simulink model "comprehensive_model_with_rocks_trial"  (R2019a)
settings: Solver=FixedStepAuto  StartTime=0.0  StopTime=15  FixedStep=0.001  RelTol=1e-3
PreLoadFcn:
  | load('tumbleweed_constants.mat')
values from neighbouring files (symbols this model uses):
  Ar = 0.785398163397    [tumbleweed_constants.mat]
  CD = 0.8    [tumbleweed_constants.mat]
  d = 0.65    [tumbleweed_constants.mat]
  g = 9.81    [tumbleweed_constants.mat]
  Ixx = 1.29    [tumbleweed_constants.mat]
  Iyy = 1.29    [tumbleweed_constants.mat]
  Izz = 1.29    [tumbleweed_constants.mat]
  m = 1    [tumbleweed_constants.mat]
  maxr = 0.45    [tumbleweed_constants.mat]
  mf = 14    [tumbleweed_constants.mat]
  minr = 0.2    [tumbleweed_constants.mat]
  mu0 = 0.02    [tumbleweed_constants.mat]
  muk = 0.5    [tumbleweed_constants.mat]
  must = 0.8    [tumbleweed_constants.mat]
  R = cylR*ones(size(Theta,1),size(Theta,2))    [d3_animate.m]    (also in tumbleweed_constants.mat = 0.5)
  rest_coeff = 0.6    [tumbleweed_constants.mat]
  rho = 1.2    [tumbleweed_constants.mat]
  ts = 0.5    [tumbleweed_constants.mat]
  v_thres = 0.0001    [tumbleweed_constants.mat]
  vmax = 0.2    [tumbleweed_constants.mat]
  YY = 50    [tumbleweed_constants.mat]
libraries: simulink x2
(part 9 of 9)

== matlab function comprehensive_model_with_rocks_trial/bouncing_model1/onsurface_model/Subsystem/MATLAB Function2 ==
  data: A21 output size=[3, 3]; t input; states input; u input; O_c_A input; O_w_A input; O_v_AO input; FW input; par_diffs input; flag input; A22 output size=[3, 3]; B2 output size=3; OalA_coeffs output size=[3,3]; OalA_consts output size=3; R parameter; g parameter; Ixx parameter; Iyy parameter; Izz parameter; m parameter; mf parameter; mu0 parameter; must parameter; d parameter; YY parameter; muk parameter; v_thres parameter
function [A21, A22, B2, OalA_coeffs, OalA_consts] = dynamics_mat_gen(t, states,u, O_c_A, O_w_A, O_v_AO, FW, par_diffs,flag, R, g, Ixx, Iyy, Izz, m, mf, mu0, must, d, YY, muk, v_thres)

y = states;
I_T = [Ixx,0,0;0,Iyy,0;0,0,Izz]; 
r_m1T = [u(1);0;0]; T_v_m1T = [u(7);0;0]; T_a_m1T = [u(13);0;0];
r_m2T = [u(2);0;0]; T_v_m2T = [u(8);0;0]; T_a_m2T = [u(14);0;0];
r_m3T = [0;u(3);0]; T_v_m3T = [0;u(9);0]; T_a_m3T = [0;u(15);0];
r_m4T = [0;u(4);0]; T_v_m4T = [0;u(10);0]; T_a_m4T = [0;u(16);0];
r_m5T = [0;0;u(5)]; T_v_m5T = [0;0;u(11)]; T_a_m5T = [0;0;u(17)];
r_m6T = [0;0;u(6)]; T_v_m6T = [0;0;u(12)]; T_a_m6T = [0;0;u(18)];
r_CMT = m*(r_m1T + r_m2T + r_m3T + r_m4T + r_m5T + r_m6T)/(6*m+mf);
T_v_CMT = m*(T_v_m1T + T_v_m2T + T_v_m3T + T_v_m4T + T_v_m5T + T_v_m6T)/(6*m+mf);
T_a_CMT = m*(T_a_m1T + T_a_m2T + T_a_m3T + T_a_m4T + T_a_m5T + T_a_m6T)/(6*m+mf);
r_CMTx = Vx(r_CMT);r_m1Tx = Vx(r_m1T);r_m2Tx = Vx(r_m2T);r_m3Tx = Vx(r_m3T);
r_m4Tx = Vx(r_m4T);r_m5Tx = Vx(r_m5T);r_m6Tx = Vx(r_m6T);
q0 = y(10);q1=y(11);q2=y(12);q3=y(13);
T_c_O = [q0^2 + q1^2 - q2^2 - q3^2, 2*(q1*q2 + q0*q3), 2*(q1*q3 - q0*q2);...
       2*(q1*q2 - q0*q3), q0^2 - q1^2 + q2^2 - q3^2, 2*(q2*q3 + q0*q1);...
       2*(q1*q3 + q0*q2), 2*(q2*q3 - q0*q1), q0^2 - q1^2 - q2^2 + q3^2];
O_c_T = T_c_O.';
T_c_A = T_c_O*O_c_A;
A_c_O = transpose(O_c_A);
A_c_T = T_c_A';
r_AT = [0;0;-R]; r_TA = [0;0;R]; r_ATx = Vx(r_AT); r_TAx = Vx(r_TA);

O_w_T = [y(1);y(2);y(3)];
A_w_T = O_w_T - T_c_A*O_w_A;
O_w_Tx = Vx(O_w_T);
O_w_Ax = Vx(O_w_A);

O_vel_TO = A_c_O*O_v_AO + cross(O_w_A, r_TA);
u_TO = O_vel_TO(1);
v_TO = O_vel_TO(2);
w_TO = O_vel_TO(3);

%mu0 =0.02;% 0.02;
murr = mu0*tanh(sqrt(u_TO^2 + v_TO^2 + w_TO^2)/v_thres); 
roll_rest_coeff = [1,0,-murr*u_TO/sqrt(u_TO^2 + v_TO^2);0,1,-murr*v_TO/sqrt(u_TO^2 + v_TO^2);0,0,1];
FG = [0;0;-(mf+6*m)*g];
FGA = A_c_O*FG;
FR  = -murr*norm(FGA'*[0;0;1])*[u_TO; v_TO; w_TO]/sqrt(u_TO^2 + v_TO^2 + w_TO^2);

eps = 0.025;
N = norm(FGA'*[0;0;1]);
f = 0.5;%0.5;
OwTz = (A_c_T*O_w_T)'*[0;0;1];
if(abs(OwTz) <= 1e-4)
    MzT = [0;0;0];
else
MzT = [0;0;-3*pi*N*f*eps*OwTz/(16*norm(OwTz))];%-mu*N*[0;0;1];
end


x_dot = O_v_AO(1);
y_dot = O_v_AO(2);
z_dot = O_v_AO(3);

fx = par_diffs(1);
fy = par_diffs(2);
fz = par_diffs(3);
fxx = par_diffs(4);
fxy = par_diffs(5);
fxz = par_diffs(6);
fyy = par_diffs(7);
fyz = par_diffs(8);
fzz = par_diffs(9);
fxxx = par_diffs(10);
fxxy = par_diffs(11);
fxxz = par_diffs(12);
fxyy = par_diffs(13);
fxyz = par_diffs(14);
fxzz = par_diffs(15);
fyyy = par_diffs(16);
fyyz = par_diffs(17);
fyzz = par_diffs(18);
fzzz = par_diffs(19);






if flag == 1
OalA_coeffs = ...
[(-(fx*fxy - fxx*fy)/((fx^2 + fy^2)^(1/2)*(fx^2 + fy^2 + fz^2)^(1/2))),                               (-(fx*fyy - fxy*fy)/((fx^2 + fy^2)^(1/2)*(fx^2 + fy^2 + fz^2)^(1/2))),                                     (-(fx*fyz - fxz*fy)/((fx^2 + fy^2)^(1/2)*(fx^2 + fy^2 + fz^2)^(1/2)));...
 (-(fxz*fx^2 - fxx*fz*fx + fxz*fy^2 - fxy*fz*fy)/((fx^2 + fy^2)^(1/2)*(fx^2 + fy^2 + fz^2))),          (-(fyz*fx^2 - fxy*fz*fx + fyz*fy^2 - fyy*fz*fy)/((fx^2 + fy^2)^(1/2)*(fx^2 + fy^2 + fz^2))),               (-(fzz*fx^2 - fxz*fz*fx + fzz*fy^2 - fyz*fz*fy)/((fx^2 + fy^2)^(1/2)*(fx^2 + fy^2 + fz^2)));...
 ((fz*(fx*fxy - fxx*fy))/((fx^2 + fy^2)*(fx^2 + fy^2 + fz^2)^(1/2))),                                  ((fz*(fx*fyy - fxy*fy))/((fx^2 + fy^2)*(fx^2 + fy^2 + fz^2)^(1/2))),                                       ((fz*(fx*fyz - fxz*fy))/((fx^2 + fy^2)*(fx^2 + fy^2 + fz^2)^(1/2)))];

OalA_consts = ...
 [((fx*(2*fxx*x_dot + 2*fxy*y_dot + 2*fxz*z_dot) + fy*(2*fxy*x_dot + 2*fyy*y_dot + 2*fyz*z_dot) + fz*(2*fxz*x_dot + 2*fyz*y_dot + 2*fzz*z_dot))*(fx*fxy*x_dot - fxx*fy*x_dot + fx*fyy*y_dot - fxy*fy*y_dot + fx*fyz*z_dot - fxz*fy*z_dot))/(2*(fx^2 + fy^2)^(1/2)*(fx^2 + fy^2 + fz^2)^(3/2)) - (fx*fxxy*x_dot^2 - fxxx*fy*x_dot^2 + fx*fyyy*y_dot^2 - fxyy*fy*y_dot^2 + fx*fyzz*z_dot^2 - fxzz*fy*z_dot^2 + 2*fx*fxyy*x_dot*y_dot - 2*fxxy*fy*x_dot*y_dot + 2*fx*fxyz*x_dot*z_dot - 2*fxxz*fy*x_dot*z_dot + 2*fx*fyyz*y_dot*z_dot - 2*fxyz*fy*y_dot*z_dot)/((fx^2 + fy^2)^(1/2)*(fx^2 + fy^2 + fz^2)^(1/2)) + ((fx*(2*fxx*x_dot + 2*fxy*y_dot + 2*fxz*z_dot) + fy*(2*fxy*x_dot + 2*fyy*y_dot + 2*fyz*z_dot))*(fx*fxy*x_dot - fxx*fy*x_dot + fx*fyy*y_dot - fxy*fy*y_dot + fx*fyz*z_dot - fxz*fy*z_dot))/(2*(fx^2 + fy^2)^(3/2)*(fx^2 + fy^2 + fz^2)^(1/2));...
 ((fx*(2*fxx*x_dot + 2*fxy*y_dot + 2*fxz*z_dot) + fy*(2*fxy*x_dot + 2*fyy*y_dot + 2*fyz*z_dot) + fz*(2*fxz*x_dot + 2*fyz*y_dot + 2*fzz*z_dot))*(fx^2*fxz*x_dot + fxz*fy^2*x_dot + fx^2*fyz*y_dot + fy^2*fyz*y_dot + fx^2*fzz*z_dot + fy^2*fzz*z_dot - fx*fxx*fz*x_dot - fxy*fy*fz*x_dot - fx*fxy*fz*y_dot - fy*fyy*fz*y_dot - fx*fxz*fz*z_dot - fy*fyz*fz*z_dot))/((fx^2 + fy^2)^(1/2)*(fx^2 + fy^2 + fz^2)^2) - (fxxz*fx^2*x_dot^2 + 2*fxyz*fx^2*x_dot*y_dot + 2*fxzz*fx^2*x_dot*z_dot + fyyz*fx^2*y_dot^2 + 2*fyzz*fx^2*y_dot*z_dot + fzzz*fx^2*z_dot^2 + fx*fxx*fxz*x_dot^2 + fx*fxx*fyz*x_dot*y_dot + fzz*fx*fxx*x_dot*z_dot + fx*fxy*fxz*x_dot*y_dot + fx*fxy*fyz*y_dot^2 + fzz*fx*fxy*y_dot*z_dot + fx*fxz^2*x_dot*z_dot + fx*fxz*fyz*y_dot*z_dot + fzz*fx*fxz*z_dot^2 - fxxx*fz*fx*x_dot^2 - 2*fxxy*fz*fx*x_dot*y_dot - 2*fxxz*fz*fx*x_dot*z_dot - fxyy*fz*fx*y_dot^2 - 2*fxyz*fz*fx*y_dot*z_dot - fxzz*fz*fx*z_dot^2 - fz*fxx^2*x_dot^2 - 2*fz*fxx*fxy*x_dot*y_dot - 2*fz*fxx*fxz*x_dot*z_dot - fz*fxy^2*x_dot^2 - fz*fxy^2*y_dot^2 + fxy*fxz*fy*x_dot^2 - 2*fz*fxy*fxz*y_dot*z_dot + fxy*fy*fyz*x_dot*y_dot + fzz*fxy*fy*x_dot*z_dot - 2*fz*fxy*fyy*x_dot*y_dot - 2*fz*fxy*fyz*x_dot*z_dot - fz*fxz^2*z_dot^2 + fxz*fy*fyy*x_dot*y_dot + fxz*fy*fyz*x_dot*z_dot + fxxz*fy^2*x_dot^2 + 2*fxyz*fy^2*x_dot*y_dot + 2*fxzz*fy^2*x_dot*z_dot + fyyz*fy^2*y_dot^2 + 2*fyzz*fy^2*y_dot*z_dot + fzzz*fy^2*z_dot^2 + fy*fyy*fyz*y_dot^2 + fzz*fy*fyy*y_dot*z_dot + fy*fyz^2*y_dot*z_dot + fzz*fy*fyz*z_dot^2 - fxxy*fz*fy*x_dot^2 - 2*fxyy*fz*fy*x_dot*y_dot - 2*fxyz*fz*fy*x_dot*z_dot - fyyy*fz*fy*y_dot^2 - 2*fyyz*fz*fy*y_dot*z_dot - fyzz*fz*fy*z_dot^2 - fz*fyy^2*y_dot^2 - 2*fz*fyy*fyz*y_dot*z_dot - fz*fyz^2*z_dot^2)/((fx^2 + fy^2)^(1/2)*(fx^2 + fy^2 + fz^2)) + ((fx*(2*fxx*x_dot + 2*fxy*y_dot + 2*fxz*z_dot) + fy*(2*fxy*x_dot + 2*fyy*y_dot + 2*fyz*z_dot))*(fx^2*fxz*x_dot + fxz*fy^2*x_dot + fx^2*fyz*y_dot + fy^2*fyz*y_dot + fx^2*fzz*z_dot + fy^2*fzz*z_dot - fx*fxx*fz*x_dot - fxy*fy*fz*x_dot - fx*fxy*fz*y_dot - fy*fyy*fz*y_dot - fx*fxz*fz*z_dot - fy*fyz*fz*z_dot))/(2*(fx^2 + fy^2)^(3/2)*(fx^2 + fy^2 + fz^2));...
 ((fxz*x_dot + fyz*y_dot + fzz*z_dot)*(fx*fxy*x_dot - fxx*fy*x_dot + fx*fyy*y_dot - fxy*fy*y_dot + fx*fyz*z_dot - fxz*fy*z_dot))/((fx^2 + fy^2)*(fx^2 + fy^2 + fz^2)^(1/2)) + (fz*(fx*fxxy*x_dot^2 - fxxx*fy*x_dot^2 + fx*fyyy*y_dot^2 - fxyy*fy*y_dot^2 + fx*fyzz*z_dot^2 - fxzz*fy*z_dot^2 + 2*fx*fxyy*x_dot*y_dot - 2*fxxy*fy*x_dot*y_dot + 2*fx*fxyz*x_dot*z_dot - 2*fxxz*fy*x_dot*z_dot + 2*fx*fyyz*y_dot*z_dot - 2*fxyz*fy*y_dot*z_dot))/((fx^2 + fy^2)*(fx^2 + fy^2 + fz^2)^(1/2)) - (fz*(fx*(2*fxx*x_dot + 2*fxy*y_dot + 2*fxz*z_dot) + fy*(2*fxy*x_dot + 2*fyy*y_dot + 2*fyz*z_dot) + fz*(2*fxz*x_dot + 2*fyz*y_dot + 2*fzz*z_dot))*(fx*fxy*x_dot - fxx*fy*x_dot + fx*fyy*y_dot - fxy*fy*y_dot + fx*fyz*z_dot - fxz*fy*z_dot))/((2*fx^2 + 2*fy^2)*(fx^2 + fy^2 + fz^2)^(3/2)) - (fz*(fx*(2*fxx*x_dot + 2*fxy*y_dot + 2*fxz*z_dot) + fy*(2*fxy*x_dot + 2*fyy*y_dot + 2*fyz*z_dot))*(fx*fxy*x_dot - fxx*fy*x_dot + fx*fyy*y_dot - fxy*fy*y_dot + fx*fyz*z_dot - fxz*fy*z_dot))/((fx^2 + fy^2)^2*(fx^2 + fy^2 + fz^2)^(1/2))];

else
    
OalA_coeffs = ...    
[((fx*fxy - fxx*fy)/((fx^2 + fy^2)^(1/2)*(fx^2 + fy^2 + fz^2)^(1/2))),                                ((fx*fyy - fxy*fy)/((fx^2 + fy^2)^(1/2)*(fx^2 + fy^2 + fz^2)^(1/2))),                                        ((fx*fyz - fxz*fy)/((fx^2 + fy^2)^(1/2)*(fx^2 + fy^2 + fz^2)^(1/2)));...
((fxz*fx^2 - fxx*fz*fx + fxz*fy^2 - fxy*fz*fy)/((fx^2 + fy^2)^(1/2)*(fx^2 + fy^2 + fz^2))),            ((fyz*fx^2 - fxy*fz*fx + fyz*fy^2 - fyy*fz*fy)/((fx^2 + fy^2)^(1/2)*(fx^2 + fy^2 + fz^2))),                  ((fzz*fx^2 - fxz*fz*fx + fzz*fy^2 - fyz*fz*fy)/((fx^2 + fy^2)^(1/2)*(fx^2 + fy^2 + fz^2)));...
((fz*(fx*fxy - fxx*fy))/((fx^2 + fy^2)*(fx^2 + fy^2 + fz^2)^(1/2))),                                   ((fz*(fx*fyy - fxy*fy))/((fx^2 + fy^2)*(fx^2 + fy^2 + fz^2)^(1/2))),                                         ((fz*(fx*fyz - fxz*fy))/((fx^2 + fy^2)*(fx^2 + fy^2 + fz^2)^(1/2)))];
    
OalA_consts = ...
[(fx*fxxy*x_dot^2 - fxxx*fy*x_dot^2 + fx*fyyy*y_dot^2 - fxyy*fy*y_dot^2 + fx*fyzz*z_dot^2 - fxzz*fy*z_dot^2 + 2*fx*fxyy*x_dot*y_dot - 2*fxxy*fy*x_dot*y_dot + 2*fx*fxyz*x_dot*z_dot - 2*fxxz*fy*x_dot*z_dot + 2*fx*fyyz*y_dot*z_dot - 2*fxyz*fy*y_dot*z_dot)/((fx^2 + fy^2)^(1/2)*(fx^2 + fy^2 + fz^2)^(1/2)) - ((fx*(2*fxx*x_dot + 2*fxy*y_dot + 2*fxz*z_dot) + fy*(2*fxy*x_dot + 2*fyy*y_dot + 2*fyz*z_dot) + fz*(2*fxz*x_dot + 2*fyz*y_dot + 2*fzz*z_dot))*(fx*fxy*x_dot - fxx*fy*x_dot + fx*fyy*y_dot - fxy*fy*y_dot + fx*fyz*z_dot - fxz*fy*z_dot))/(2*(fx^2 + fy^2)^(1/2)*(fx^2 + fy^2 + fz^2)^(3/2)) - ((fx*(2*fxx*x_dot + 2*fxy*y_dot + 2*fxz*z_dot) + fy*(2*fxy*x_dot + 2*fyy*y_dot + 2*fyz*z_dot))*(fx*fxy*x_dot - fxx*fy*x_dot + fx*fyy*y_dot - fxy*fy*y_dot + fx*fyz*z_dot - fxz*fy*z_dot))/(2*(fx^2 + fy^2)^(3/2)*(fx^2 + fy^2 + fz^2)^(1/2));...
 (fxxz*fx^2*x_dot^2 + 2*fxyz*fx^2*x_dot*y_dot + 2*fxzz*fx^2*x_dot*z_dot + fyyz*fx^2*y_dot^2 + 2*fyzz*fx^2*y_dot*z_dot + fzzz*fx^2*z_dot^2 + fx*fxx*fxz*x_dot^2 + fx*fxx*fyz*x_dot*y_dot + fzz*fx*fxx*x_dot*z_dot + fx*fxy*fxz*x_dot*y_dot + fx*fxy*fyz*y_dot^2 + fzz*fx*fxy*y_dot*z_dot + fx*fxz^2*x_dot*z_dot + fx*fxz*fyz*y_dot*z_dot + fzz*fx*fxz*z_dot^2 - fxxx*fz*fx*x_dot^2 - 2*fxxy*fz*fx*x_dot*y_dot - 2*fxxz*fz*fx*x_dot*z_dot - fxyy*fz*fx*y_dot^2 - 2*fxyz*fz*fx*y_dot*z_dot - fxzz*fz*fx*z_dot^2 - fz*fxx^2*x_dot^2 - 2*fz*fxx*fxy*x_dot*y_dot - 2*fz*fxx*fxz*x_dot*z_dot - fz*fxy^2*x_dot^2 - fz*fxy^2*y_dot^2 + fxy*fxz*fy*x_dot^2 - 2*fz*fxy*fxz*y_dot*z_dot + fxy*fy*fyz*x_dot*y_dot + fzz*fxy*fy*x_dot*z_dot - 2*fz*fxy*fyy*x_dot*y_dot - 2*fz*fxy*fyz*x_dot*z_dot - fz*fxz^2*z_dot^2 + fxz*fy*fyy*x_dot*y_dot + fxz*fy*fyz*x_dot*z_dot + fxxz*fy^2*x_dot^2 + 2*fxyz*fy^2*x_dot*y_dot + 2*fxzz*fy^2*x_dot*z_dot + fyyz*fy^2*y_dot^2 + 2*fyzz*fy^2*y_dot*z_dot + fzzz*fy^2*z_dot^2 + fy*fyy*fyz*y_dot^2 + fzz*fy*fyy*y_dot*z_dot + fy*fyz^2*y_dot*z_dot + fzz*fy*fyz*z_dot^2 - fxxy*fz*fy*x_dot^2 - 2*fxyy*fz*fy*x_dot*y_dot - 2*fxyz*fz*fy*x_dot*z_dot - fyyy*fz*fy*y_dot^2 - 2*fyyz*fz*fy*y_dot*z_dot - fyzz*fz*fy*z_dot^2 - fz*fyy^2*y_dot^2 - 2*fz*fyy*fyz*y_dot*z_dot - fz*fyz^2*z_dot^2)/((fx^2 + fy^2)^(1/2)*(fx^2 + fy^2 + fz^2)) - ((fx*(2*fxx*x_dot + 2*fxy*y_dot + 2*fxz*z_dot) + fy*(2*fxy*x_dot + 2*fyy*y_dot + 2*fyz*z_dot) + fz*(2*fxz*x_dot + 2*fyz*y_dot + 2*fzz*z_dot))*(fx^2*fxz*x_dot + fxz*fy^2*x_dot + fx^2*fyz*y_dot + fy^2*fyz*y_dot + fx^2*fzz*z_dot + fy^2*fzz*z_dot - fx*fxx*fz*x_dot - fxy*fy*fz*x_dot - fx*fxy*fz*y_dot - fy*fyy*fz*y_dot - fx*fxz*fz*z_dot - fy*fyz*fz*z_dot))/((fx^2 + fy^2)^(1/2)*(fx^2 + fy^2 + fz^2)^2) - ((fx*(2*fxx*x_dot + 2*fxy*y_dot + 2*fxz*z_dot) + fy*(2*fxy*x_dot + 2*fyy*y_dot + 2*fyz*z_dot))*(fx^2*fxz*x_dot + fxz*fy^2*x_dot + fx^2*fyz*y_dot + fy^2*fyz*y_dot + fx^2*fzz*z_dot + fy^2*fzz*z_dot - fx*fxx*fz*x_dot - fxy*fy*fz*x_dot - fx*fxy*fz*y_dot - fy*fyy*fz*y_dot - fx*fxz*fz*z_dot - fy*fyz*fz*z_dot))/(2*(fx^2 + fy^2)^(3/2)*(fx^2 + fy^2 + fz^2));...
 ((fxz*x_dot + fyz*y_dot + fzz*z_dot)*(fx*fxy*x_dot - fxx*fy*x_dot + fx*fyy*y_dot - fxy*fy*y_dot + fx*fyz*z_dot - fxz*fy*z_dot))/((fx^2 + fy^2)*(fx^2 + fy^2 + fz^2)^(1/2)) + (fz*(fx*fxxy*x_dot^2 - fxxx*fy*x_dot^2 + fx*fyyy*y_dot^2 - fxyy*fy*y_dot^2 + fx*fyzz*z_dot^2 - fxzz*fy*z_dot^2 + 2*fx*fxyy*x_dot*y_dot - 2*fxxy*fy*x_dot*y_dot + 2*fx*fxyz*x_dot*z_dot - 2*fxxz*fy*x_dot*z_dot + 2*fx*fyyz*y_dot*z_dot - 2*fxyz*fy*y_dot*z_dot))/((fx^2 + fy^2)*(fx^2 + fy^2 + fz^2)^(1/2)) - (fz*(fx*(2*fxx*x_dot + 2*fxy*y_dot + 2*fxz*z_dot) + fy*(2*fxy*x_dot + 2*fyy*y_dot + 2*fyz*z_dot) + fz*(2*fxz*x_dot + 2*fyz*y_dot + 2*fzz*z_dot))*(fx*fxy*x_dot - fxx*fy*x_dot + fx*fyy*y_dot - fxy*fy*y_dot + fx*fyz*z_dot - fxz*fy*z_dot))/((2*fx^2 + 2*fy^2)*(fx^2 + fy^2 + fz^2)^(3/2)) - (fz*(fx*(2*fxx*x_dot + 2*fxy*y_dot + 2*fxz*z_dot) + fy*(2*fxy*x_dot + 2*fyy*y_dot + 2*fyz*z_dot))*(fx*fxy*x_dot - fxx*fy*x_dot + fx*fyy*y_dot - fxy*fy*y_dot + fx*fyz*z_dot - fxz*fy*z_dot))/((fx^2 + fy^2)^2*(fx^2 + fy^2 + fz^2)^(1/2))];
 
end    

if abs(fx) <= 1e-20 && abs(fy) <= 1e-20
    OalA_coeffs = zeros(3,3);
    OalA_consts  = zeros(3,1);
end

A21 = I_T + (mf + 6*m)*T_c_A*r_ATx*A_c_T*r_CMTx - m*r_m1Tx*r_m1Tx - m*r_m2Tx*r_m2Tx...
       - m*r_m3Tx*r_m3Tx - m*r_m4Tx*r_m4Tx - m*r_m5Tx*r_m5Tx - m*r_m6Tx*r_m6Tx;
   
A22 = (mf + 6*m)*r_CMTx*T_c_A*(A_c_O - r_TAx*OalA_coeffs) +  ...
      (mf + 6*m)*T_c_A*r_TAx*(A_c_O - r_TAx*OalA_coeffs);
  
  
B2 = -cross(O_w_T,I_T*O_w_T) - m*cross(r_m1T,2*O_w_Tx*T_v_m1T + O_w_Tx*O_w_Tx*r_m1T)...
       - m*r_m2Tx*(T_a_m2T + 2*O_w_Tx*T_v_m2T + O_w_Tx*O_w_Tx*r_m2T)...
       - m*r_m3Tx*(T_a_m3T + 2*O_w_Tx*T_v_m3T + O_w_Tx*O_w_Tx*r_m3T)...
       - m*r_m4Tx*(T_a_m4T + 2*O_w_Tx*T_v_m4T + O_w_Tx*O_w_Tx*r_m4T)...
       - m*r_m5Tx*(T_a_m5T + 2*O_w_Tx*T_v_m5T + O_w_Tx*O_w_Tx*r_m5T)...
       - m*r_m6Tx*(T_a_m6T + 2*O_w_Tx*T_v_m6T + O_w_Tx*O_w_Tx*r_m6T)...
       + r_CMTx*T_c_O*FG  + (mf + 6*m)*cross(T_c_A*r_AT, T_a_CMT + ...
         2*O_w_Tx*T_v_CMT + O_w_Tx*O_w_Tx*r_CMT) - cross(T_c_A*r_AT, T_c_O*FG) ...
         - cross(T_c_A*r_AT, T_c_A*FR) - cross(T_c_A*r_AT, T_c_O*FW) + T_c_A*MzT +...
         + (mf + 6*m)*r_CMTx*T_c_A*(r_TAx*OalA_consts - O_w_Ax*O_w_Ax*r_TA)...
         + (mf + 6*m)*T_c_A*r_TAx*(r_TAx*OalA_consts - O_w_Ax*O_w_Ax*r_TA);    
end

== matlab function comprehensive_model_with_rocks_trial/bouncing_model1/onsurface_model/Subsystem/MATLAB Function3 ==
  data: t input; A11 input; angacc_linacc output size=6; A12 input; A21 input; A22 input; B1 input; B2 input
function angacc_linacc = state_solver(t,A11,A12,A21,A22,B1,B2)
if t== 0.5
    disp(t)
end
Amat = [A11,A12;A21,A22];
Bvec = [B1;B2];
 angacc_linacc = inv(Amat)*Bvec;
end

== matlab function comprehensive_model_with_rocks_trial/bouncing_model1/onsurface_model/Subsystem/MATLAB Function6 ==
  data: angacc_linacc input; states input; u input size=18; O_c_A input; O_w_A input; slip_flag output size=1; OalA_coeffs input; OalA_consts input; slip_flag0 input; FW input; mf parameter; m parameter; R parameter; must parameter; mu0 parameter; v_thres parameter; g parameter; FN output
function [slip_flag, FN] = FC_calc(angacc_linacc, states,u, O_c_A, O_w_A, OalA_coeffs, OalA_consts, slip_flag0, FW, mf, m, R, must, mu0, v_thres, g)
if slip_flag0 == false
y = states;
r_m1T = [u(1);0;0]; T_v_m1T = [u(7);0;0]; T_a_m1T = [u(13);0;0];
r_m2T = [u(2);0;0]; T_v_m2T = [u(8);0;0]; T_a_m2T = [u(14);0;0];
r_m3T = [0;u(3);0]; T_v_m3T = [0;u(9);0]; T_a_m3T = [0;u(15);0];
r_m4T = [0;u(4);0]; T_v_m4T = [0;u(10);0]; T_a_m4T = [0;u(16);0];
r_m5T = [0;0;u(5)]; T_v_m5T = [0;0;u(11)]; T_a_m5T = [0;0;u(17)];
r_m6T = [0;0;u(6)]; T_v_m6T = [0;0;u(12)]; T_a_m6T = [0;0;u(18)];
r_CMT = m*(r_m1T + r_m2T + r_m3T + r_m4T + r_m5T + r_m6T)/(6*m+mf);
T_v_CMT = m*(T_v_m1T + T_v_m2T + T_v_m3T + T_v_m4T + T_v_m5T + T_v_m6T)/(6*m+mf);
T_a_CMT = m*(T_a_m1T + T_a_m2T + T_a_m3T + T_a_m4T + T_a_m5T + T_a_m6T)/(6*m+mf);

O_w_T = [y(1);y(2);y(3)];
q0 = y(10);q1=y(11);q2=y(12);q3=y(13);
T_c_O = [q0^2 + q1^2 - q2^2 - q3^2, 2*(q1*q2 + q0*q3), 2*(q1*q3 - q0*q2);...
       2*(q1*q2 - q0*q3), q0^2 - q1^2 + q2^2 - q3^2, 2*(q2*q3 + q0*q1);...
       2*(q1*q3 + q0*q2), 2*(q2*q3 - q0*q1), q0^2 - q1^2 - q2^2 + q3^2];
O_c_T = T_c_O.';
A_c_O = O_c_A.';
r_TA = [0;0;R];
r_TAx = Vx(r_TA);
r_AT = [0;0;-R];
r_ATx = Vx(r_AT);
O_w_Ax = Vx(O_w_A);
O_al_T = [angacc_linacc(1);angacc_linacc(2);angacc_linacc(3)];
O_a_AO = [angacc_linacc(4);angacc_linacc(5);angacc_linacc(6)];

O_vel_TO = A_c_O*[states(4);states(5);states(6)];
u_TO = O_vel_TO(1);
v_TO = O_vel_TO(2);
w_TO = O_vel_TO(3);
murr = mu0*tanh(sqrt(u_TO^2 + v_TO^2 + w_TO^2)/v_thres); 
roll_rest_coeff = [1,0,-murr*u_TO/sqrt(u_TO^2 + v_TO^2);0,1,-murr*v_TO/sqrt(u_TO^2 + v_TO^2);0,0,1];
FG = [0;0;-(mf+6*m)*g];
FGA = A_c_O*FG;
FR  = -murr*norm(FGA'*[0;0;1])*[u_TO; v_TO; w_TO]/sqrt(u_TO^2 + v_TO^2 + w_TO^2);



FC = A_c_O*((mf + 6*m)*O_c_T*(T_a_CMT + cross(O_al_T,r_CMT) + 2*cross(O_w_T,T_v_CMT) + cross(O_w_T,cross(O_w_T,r_CMT))) + ...
    (mf + 6*m)*(O_a_AO - O_c_A*r_TAx*(OalA_coeffs*O_a_AO + OalA_consts) + O_c_A*O_w_Ax*O_w_Ax*r_TA) - O_c_A*FR - FG - FW);

FFRx = FC(1); FFRy = FC(2); FN = FC(3);

    if norm([FFRx;FFRy]) >= must*FN
        slip_flag = true;
    else
        slip_flag = false;
    end
else
    slip_flag = slip_flag0;
    FN = 0;
end

if slip_flag == true
    disp(slip_flag);
end
end

== matlab function comprehensive_model_with_rocks_trial/bouncing_model/onsurface_model/Subsystem/MATLAB Function3 ==
  data: t input; A11 input; angacc_linacc output size=6; A12 input; A21 input; A22 input; B1 input; B2 input
function angacc_linacc = state_solver(t,A11,A12,A21,A22,B1,B2)
if t== 0.5
    disp(t)
end
Amat = [A11,A12;A21,A22];
Bvec = [B1;B2];
 angacc_linacc = inv(Amat)*Bvec;
end

== matlab function comprehensive_model_with_rocks_trial/bouncing_model/onsurface_model/Subsystem/MATLAB Function6 ==
  data: angacc_linacc input; states input; u input size=18; O_c_A input; O_w_A input; slip_flag output size=1; OalA_coeffs input; OalA_consts input; slip_flag0 input; FW input; mf parameter; m parameter; R parameter; must parameter; mu0 parameter; v_thres parameter; g parameter; FN output
function [slip_flag, FN] = FC_calc(angacc_linacc, states,u, O_c_A, O_w_A, OalA_coeffs, OalA_consts, slip_flag0, FW, mf, m, R, must, mu0, v_thres, g)
if slip_flag0 == false
y = states;
r_m1T = [u(1);0;0]; T_v_m1T = [u(7);0;0]; T_a_m1T = [u(13);0;0];
r_m2T = [u(2);0;0]; T_v_m2T = [u(8);0;0]; T_a_m2T = [u(14);0;0];
r_m3T = [0;u(3);0]; T_v_m3T = [0;u(9);0]; T_a_m3T = [0;u(15);0];
r_m4T = [0;u(4);0]; T_v_m4T = [0;u(10);0]; T_a_m4T = [0;u(16);0];
r_m5T = [0;0;u(5)]; T_v_m5T = [0;0;u(11)]; T_a_m5T = [0;0;u(17)];
r_m6T = [0;0;u(6)]; T_v_m6T = [0;0;u(12)]; T_a_m6T = [0;0;u(18)];
r_CMT = m*(r_m1T + r_m2T + r_m3T + r_m4T + r_m5T + r_m6T)/(6*m+mf);
T_v_CMT = m*(T_v_m1T + T_v_m2T + T_v_m3T + T_v_m4T + T_v_m5T + T_v_m6T)/(6*m+mf);
T_a_CMT = m*(T_a_m1T + T_a_m2T + T_a_m3T + T_a_m4T + T_a_m5T + T_a_m6T)/(6*m+mf);

O_w_T = [y(1);y(2);y(3)];
q0 = y(10);q1=y(11);q2=y(12);q3=y(13);
T_c_O = [q0^2 + q1^2 - q2^2 - q3^2, 2*(q1*q2 + q0*q3), 2*(q1*q3 - q0*q2);...
       2*(q1*q2 - q0*q3), q0^2 - q1^2 + q2^2 - q3^2, 2*(q2*q3 + q0*q1);...
       2*(q1*q3 + q0*q2), 2*(q2*q3 - q0*q1), q0^2 - q1^2 - q2^2 + q3^2];
O_c_T = T_c_O.';
A_c_O = O_c_A.';
r_TA = [0;0;R];
r_TAx = Vx(r_TA);
r_AT = [0;0;-R];
r_ATx = Vx(r_AT);
O_w_Ax = Vx(O_w_A);
O_al_T = [angacc_linacc(1);angacc_linacc(2);angacc_linacc(3)];
O_a_AO = [angacc_linacc(4);angacc_linacc(5);angacc_linacc(6)];

O_vel_TO = A_c_O*[states(4);states(5);states(6)];
u_TO = O_vel_TO(1);
v_TO = O_vel_TO(2);
w_TO = O_vel_TO(3);
murr = mu0*tanh(sqrt(u_TO^2 + v_TO^2 + w_TO^2)/v_thres); 
roll_rest_coeff = [1,0,-murr*u_TO/sqrt(u_TO^2 + v_TO^2);0,1,-murr*v_TO/sqrt(u_TO^2 + v_TO^2);0,0,1];
FG = [0;0;-(mf+6*m)*g];
FGA = A_c_O*FG;
FR  = -murr*norm(FGA'*[0;0;1])*[u_TO; v_TO; w_TO]/sqrt(u_TO^2 + v_TO^2 + w_TO^2);



FC = A_c_O*((mf + 6*m)*O_c_T*(T_a_CMT + cross(O_al_T,r_CMT) + 2*cross(O_w_T,T_v_CMT) + cross(O_w_T,cross(O_w_T,r_CMT))) + ...
    (mf + 6*m)*(O_a_AO - O_c_A*r_TAx*(OalA_coeffs*O_a_AO + OalA_consts) + O_c_A*O_w_Ax*O_w_Ax*r_TA) - O_c_A*FR - FG - FW);

FFRx = FC(1); FFRy = FC(2); FN = FC(3);

    if norm([FFRx;FFRy]) >= must*FN
        slip_flag = true;
    else
        slip_flag = false;
    end
else
    slip_flag = slip_flag0;
    FN = 0;
end

if slip_flag == true
    disp(slip_flag);
end
end

== matlab function comprehensive_model_with_rocks_trial/nmpc1/MATLAB Function1 ==
  data: t input; udot output; rm input; udot_mat input; idx input; idx_n output; ts parameter
function [udot,idx_n] = datalookup(t,rm,udot_mat,idx,ts)
if mod(t,ts) == round(mod(t,ts))
    udot = udot_mat(1:3,idx);
    idx_n = idx +1;
else
    udot = rm(7:2:12,1);
    idx_n = idx;
end

== matlab function comprehensive_model_with_rocks_trial/nmpc1/u_dot generator ==
  data: t input size=1; states input size=13; udotc output; g parameter; Ixx parameter; Iyy parameter; Izz parameter; m parameter; mf parameter; mu0 parameter; R parameter; v_thres parameter; rm input size=18; FW input; idxn output; udot_mat input; idx input; ts parameter size=1; vmax parameter; minr parameter; maxr parameter
function [udotc,idxn] = u_dynamics(t, states,g, Ixx, Iyy, Izz, m, mf, mu0, R, v_thres, rm, FW,udot_mat,idx,ts, vmax, minr, maxr)
ts = 0.5;
upd_t = 1;
if mod(t,upd_t) == round(mod(t,upd_t))
    opthor = 2; 
    udotc = zeros(3,opthor/ts);
    udotc = nmpc_opt(opthor,t, ts, states, rm, FW,g, Ixx, Iyy, Izz, m, mf, mu0, R, v_thres, vmax, minr, maxr);
    idxn = 1;
else
    udotc = udot_mat;
    idxn = idx;
end

== matlab function comprehensive_model_with_rocks_trial/bouncing_model/MATLAB Function10 ==
  data: kA input; b1 output; states input; b2 output; R parameter
function [b1,b2] = boundary_plot(kA, states, R)
O_v_TO = states(4:6,1);
r_TO = states(7:9,1);
v1 = O_v_TO/norm(O_v_TO);
v2 = kA;
n = cross(v1,v2);
b1 = r_TO + R*n;
b2 = r_TO - R*n;
end

== matlab function comprehensive_model_with_rocks_trial/command filter based backstepper1/MATLAB Function ==
  data: t input; states input; rm input; v output size=3; wc input size=3; wc_dot input size=3; f1 input; ref input size=3; eta1 input; v_c input; FW input; v_thres parameter; d parameter; R parameter; mu0 parameter; mf parameter; m parameter; Izz parameter; Iyy parameter; Ixx parameter; g parameter; f3_v output size=3; K2 output size=[3,3]; fval output size=1; v_c output; M_hat output size=[3,3]; minr parameter size=1; maxr parameter size=1; vmax parameter
function [v,f3_v, K2,fval,v_c,M_hat]    = v_calculator(t, states, rm, wc, wc_dot, f1, ref, eta1, v_c,FW,v_thres, d, R, mu0, mf, m, Izz, Iyy, Ixx, g,minr, maxr, vmax)
x = [states(7);states(8);states(9)];
O_w_T = [states(1);states(2);states(3)]; 
if t ==55
    disp(t)
end
K2 = 0.5*eye(3);
ts = 0.01;
v = zeros(3,1);
fval = 0;
if mod(t,0.1) == 0
lhs = wc_dot - K2*(O_w_T - wc) - (f1.')*(x - ref -eta1);
%FW = [0;0;0];
[v, fval] = controlsolver(ts, lhs, states, rm, FW,g, Ixx, Iyy, Izz, m, mf, mu0, R, d, v_thres, minr, maxr);


else
    v = v_c(1:3,1);
    fval = v_c(4,1);
end
v_c = [v;fval];

I_T = [Ixx,0,0;0,Iyy,0;0,0,Izz];
r_m1T = [v(1);0;0];             T_v_m1T = [rm(7);0;0]; T_a_m1T = [rm(13);0;0];
r_m2T = [-(d - v(1));0;0];      T_v_m2T = [rm(8);0;0]; T_a_m2T = [rm(14);0;0];
r_m3T = [0;v(2);0];             T_v_m3T = [0;rm(9);0]; T_a_m3T = [0;rm(15);0];
r_m4T = [0;-(d - v(2));0];      T_v_m4T = [0;rm(10);0]; T_a_m4T = [0;rm(16);0];
r_m5T = [0;0;v(3)];             T_v_m5T = [0;0;rm(11)]; T_a_m5T = [0;0;rm(17)];
r_m6T = [0;0;-(d - v(3))];      T_v_m6T = [0;0;rm(12)]; T_a_m6T = [0;0;rm(18)];
r_CMT = m*(r_m1T + r_m2T + r_m3T + r_m4T + r_m5T + r_m6T)/(6*m+mf);
T_v_CMT = m*(T_v_m1T + T_v_m2T + T_v_m3T + T_v_m4T + T_v_m5T + T_v_m6T)/(6*m+mf);
T_a_CMT = m*(T_a_m1T + T_a_m2T + T_a_m3T + T_a_m4T + T_a_m5T + T_a_m6T)/(6*m+mf);
r_CMTx = Vx(r_CMT);r_m1Tx = Vx(r_m1T);r_m2Tx = Vx(r_m2T);r_m3Tx = Vx(r_m3T);
r_m4Tx = Vx(r_m4T);r_m5Tx = Vx(r_m5T);r_m6Tx = Vx(r_m6T);
q0 = states(10);q1=states(11);q2=states(12);q3=states(13);
T_c_O = [q0^2 + q1^2 - q2^2 - q3^2, 2*(q1*q2 + q0*q3), 2*(q1*q3 - q0*q2);...
       2*(q1*q2 - q0*q3), q0^2 - q1^2 + q2^2 - q3^2, 2*(q2*q3 + q0*q1);...
       2*(q1*q3 + q0*q2), 2*(q2*q3 - q0*q1), q0^2 - q1^2 - q2^2 + q3^2];
O_c_T = transpose(T_c_O);  
r_PT = [0;0;-R];
r_PTx = Vx([0;0;-R]);
O_w_T = [states(1);states(2);states(3)]; O_w_Tx =Vx(O_w_T);

O_vel_TO = Vx(O_c_T*O_w_T)*[0;0;R];
u_TO = O_vel_TO(1);
v_TO = O_vel_TO(2);

murr = mu0*tanh((u_TO^2 + v_TO^2)/v_thres); 
roll_rest_coeff = [1,0,-murr*u_TO/sqrt(u_TO^2 + v_TO^2);0,1,-murr*v_TO/sqrt(u_TO^2 + v_TO^2);0,0,1];
FG = [0;0;-(mf+6*m)*g];
FR  = -murr*norm(FG)/sqrt(u_TO^2 + v_TO^2)*[u_TO; v_TO; 0];

Amat = I_T + (mf + 6*m)*r_CMTx*T_c_O*r_PTx*O_c_T - m*r_m1Tx*r_m1Tx - m*r_m2Tx*r_m2Tx...
       - m*r_m3Tx*r_m3Tx - m*r_m4Tx*r_m4Tx - m*r_m5Tx*r_m5Tx - m*r_m6Tx*r_m6Tx...
       - (mf + 6*m)*Vx(T_c_O*r_PT)*Vx(T_c_O*r_PT) + (mf + 6*m)*Vx(T_c_O*r_PT)*r_CMTx;
  %some mistakes here. check again 
Bvec = -cross(O_w_T,I_T*O_w_T) - m*cross(r_m1T,2*O_w_Tx*T_v_m1T + O_w_Tx*O_w_Tx*r_m1T)...
       - m*r_m2Tx*(T_a_m2T + 2*O_w_Tx*T_v_m2T + O_w_Tx*O_w_Tx*r_m2T)...
       - m*r_m3Tx*(T_a_m3T + 2*O_w_Tx*T_v_m3T + O_w_Tx*O_w_Tx*r_m3T)...
       - m*r_m4Tx*(T_a_m4T + 2*O_w_Tx*T_v_m4T + O_w_Tx*O_w_Tx*r_m4T)...
       - m*r_m5Tx*(T_a_m5T + 2*O_w_Tx*T_v_m5T + O_w_Tx*O_w_Tx*r_m5T)...
       - m*r_m6Tx*(T_a_m6T + 2*O_w_Tx*T_v_m6T + O_w_Tx*O_w_Tx*r_m6T)...
       + r_CMTx*T_c_O*FG + (mf + 6*m)*cross(T_c_O*r_PT, T_a_CMT + ...
         2*O_w_Tx*T_v_CMT + O_w_Tx*O_w_Tx*r_CMT) - T_c_O*cross(r_PT, FG) ...
        - T_c_O*cross(r_PT, FW);%- T_c_O*cross(r_PT, FR);
f3_v = inv(Amat)*Bvec;
M_hat = inv(Amat);

end

== matlab function comprehensive_model_with_rocks_trial/command filter based backstepper1/MATLAB Function1 ==
  data: eta1 input; eta1_dot output; eta2 input; alpha input; wc input; f1 input; K1 input
function eta1_dot = eta1_dot_calc(eta1, eta2, alpha, wc, f1, K1)
eta1_dot = -K1*(eta1) + f1*(wc - alpha) + f1*eta2;
end

== matlab function comprehensive_model_with_rocks_trial/command filter based backstepper1/MATLAB Function2 ==
  data: eta2 input; K2 input; f3_v input; f3_u input; eta2_dot output
function eta2_dot = eta2_dot_calc(eta2, K2,f3_v, f3_u)
eta2_dot = -K2*eta2 + (f3_u - f3_v);
end

== matlab function comprehensive_model_with_rocks_trial/command filter based backstepper1/Subsystem/MATLAB Function ==
  data: u input; f3_u output size=3; u_dot input; u_ddot input; states input; v_thres parameter; d parameter; R parameter; mu0 parameter; mf parameter; m parameter; Izz parameter; Iyy parameter; Ixx parameter; g parameter
function f3_u = f3u_calculator(u,u_dot,u_ddot,states,v_thres, d, R, mu0, mf, m, Izz, Iyy, Ixx, g)
I_T = [Ixx,0,0;0,Iyy,0;0,0,Izz];
r_m1T = [u(1);0;0];             T_v_m1T = [u_dot(1);0;0]; T_a_m1T = [u_ddot(1);0;0];
r_m2T = [-(d - u(1));0;0];      T_v_m2T = [u_dot(1);0;0]; T_a_m2T = [u_ddot(1);0;0];
r_m3T = [0;u(2);0];             T_v_m3T = [0;u_dot(2);0]; T_a_m3T = [0;u_ddot(2);0];
r_m4T = [0;-(d - u(2));0];      T_v_m4T = [0;u_dot(2);0]; T_a_m4T = [0;u_ddot(2);0];
r_m5T = [0;0;u(3)];             T_v_m5T = [0;0;u_dot(3)]; T_a_m5T = [0;0;u_ddot(3)];
r_m6T = [0;0;-(d - u(3))];      T_v_m6T = [0;0;u_dot(3)]; T_a_m6T = [0;0;u_ddot(3)];
r_CMT = m*(r_m1T + r_m2T + r_m3T + r_m4T + r_m5T + r_m6T)/(6*m+mf);
T_v_CMT = m*(T_v_m1T + T_v_m2T + T_v_m3T + T_v_m4T + T_v_m5T + T_v_m6T)/(6*m+mf);
T_a_CMT = m*(T_a_m1T + T_a_m2T + T_a_m3T + T_a_m4T + T_a_m5T + T_a_m6T)/(6*m+mf);
r_CMTx = Vx(r_CMT);r_m1Tx = Vx(r_m1T);r_m2Tx = Vx(r_m2T);r_m3Tx = Vx(r_m3T);
r_m4Tx = Vx(r_m4T);r_m5Tx = Vx(r_m5T);r_m6Tx = Vx(r_m6T);
q0 = states(10);q1=states(11);q2=states(12);q3=states(13);
T_c_O = [q0^2 + q1^2 - q2^2 - q3^2, 2*(q1*q2 + q0*q3), 2*(q1*q3 - q0*q2);...
       2*(q1*q2 - q0*q3), q0^2 - q1^2 + q2^2 - q3^2, 2*(q2*q3 + q0*q1);...
       2*(q1*q3 + q0*q2), 2*(q2*q3 - q0*q1), q0^2 - q1^2 - q2^2 + q3^2];
O_c_T = transpose(T_c_O);  
r_PT = [0;0;-R];
r_PTx = Vx([0;0;-R]);
O_w_T = [states(1);states(2);states(3)]; O_w_Tx =Vx(O_w_T);

O_vel_TO = Vx(O_c_T*O_w_T)*[0;0;R];
u_TO = O_vel_TO(1);
v_TO = O_vel_TO(2);

murr = mu0*tanh((u_TO^2 + v_TO^2)/v_thres); 
roll_rest_coeff = [1,0,-murr*u_TO/sqrt(u_TO^2 + v_TO^2);0,1,-murr*v_TO/sqrt(u_TO^2 + v_TO^2);0,0,1];
FG = [0;0;-(mf+6*m)*g];
FR  = -murr*norm(FG)/sqrt(u_TO^2 + v_TO^2)*[u_TO; v_TO; 0];

f3_u = zeros(3,1);
Amat = I_T + (mf + 6*m)*r_CMTx*T_c_O*r_PTx*O_c_T - m*r_m1Tx*r_m1Tx - m*r_m2Tx*r_m2Tx...
       - m*r_m3Tx*r_m3Tx - m*r_m4Tx*r_m4Tx - m*r_m5Tx*r_m5Tx - m*r_m6Tx*r_m6Tx...
       - (mf + 6*m)*Vx(T_c_O*r_PT)*Vx(T_c_O*r_PT) + (mf + 6*m)*Vx(T_c_O*r_PT)*r_CMTx;
  %some mistakes here. check again 
Bvec = -cross(O_w_T,I_T*O_w_T) - m*cross(r_m1T,2*O_w_Tx*T_v_m1T + O_w_Tx*O_w_Tx*r_m1T)...
       - m*r_m2Tx*(T_a_m2T + 2*O_w_Tx*T_v_m2T + O_w_Tx*O_w_Tx*r_m2T)...
       - m*r_m3Tx*(T_a_m3T + 2*O_w_Tx*T_v_m3T + O_w_Tx*O_w_Tx*r_m3T)...
       - m*r_m4Tx*(T_a_m4T + 2*O_w_Tx*T_v_m4T + O_w_Tx*O_w_Tx*r_m4T)...
       - m*r_m5Tx*(T_a_m5T + 2*O_w_Tx*T_v_m5T + O_w_Tx*O_w_Tx*r_m5T)...
       - m*r_m6Tx*(T_a_m6T + 2*O_w_Tx*T_v_m6T + O_w_Tx*O_w_Tx*r_m6T)...
       + r_CMTx*T_c_O*FG + (mf + 6*m)*cross(T_c_O*r_PT, T_a_CMT + ...
         2*O_w_Tx*T_v_CMT + O_w_Tx*O_w_Tx*r_CMT) - T_c_O*cross(r_PT, FG) ...
         - T_c_O*cross(r_PT, FR);
f3_u = inv(Amat)*Bvec;
end

== matlab function comprehensive_model_with_rocks_trial/command filter based backstepper1/Subsystem1/MATLAB Function ==
  data: u input; f3_u output size=3; u_dot input; u_ddot input; states input; FW input; v_thres parameter; d parameter; R parameter; mu0 parameter; mf parameter; m parameter; Izz parameter; Iyy parameter; Ixx parameter; g parameter
function f3_u = f3u_calculator(u,u_dot,u_ddot,states,FW,v_thres, d, R, mu0, mf, m, Izz, Iyy, Ixx, g)
I_T = [Ixx,0,0;0,Iyy,0;0,0,Izz];
r_m1T = [u(1);0;0];             T_v_m1T = [u_dot(1);0;0]; T_a_m1T = [u_ddot(1);0;0];
r_m2T = [-(d - u(1));0;0];      T_v_m2T = [u_dot(1);0;0]; T_a_m2T = [u_ddot(1);0;0];
r_m3T = [0;u(2);0];             T_v_m3T = [0;u_dot(2);0]; T_a_m3T = [0;u_ddot(2);0];
r_m4T = [0;-(d - u(2));0];      T_v_m4T = [0;u_dot(2);0]; T_a_m4T = [0;u_ddot(2);0];
r_m5T = [0;0;u(3)];             T_v_m5T = [0;0;u_dot(3)]; T_a_m5T = [0;0;u_ddot(3)];
r_m6T = [0;0;-(d - u(3))];      T_v_m6T = [0;0;u_dot(3)]; T_a_m6T = [0;0;u_ddot(3)];
r_CMT = m*(r_m1T + r_m2T + r_m3T + r_m4T + r_m5T + r_m6T)/(6*m+mf);
T_v_CMT = m*(T_v_m1T + T_v_m2T + T_v_m3T + T_v_m4T + T_v_m5T + T_v_m6T)/(6*m+mf);
T_a_CMT = m*(T_a_m1T + T_a_m2T + T_a_m3T + T_a_m4T + T_a_m5T + T_a_m6T)/(6*m+mf);
r_CMTx = Vx(r_CMT);r_m1Tx = Vx(r_m1T);r_m2Tx = Vx(r_m2T);r_m3Tx = Vx(r_m3T);
r_m4Tx = Vx(r_m4T);r_m5Tx = Vx(r_m5T);r_m6Tx = Vx(r_m6T);
q0 = states(10);q1=states(11);q2=states(12);q3=states(13);
T_c_O = [q0^2 + q1^2 - q2^2 - q3^2, 2*(q1*q2 + q0*q3), 2*(q1*q3 - q0*q2);...
       2*(q1*q2 - q0*q3), q0^2 - q1^2 + q2^2 - q3^2, 2*(q2*q3 + q0*q1);...
       2*(q1*q3 + q0*q2), 2*(q2*q3 - q0*q1), q0^2 - q1^2 - q2^2 + q3^2];
O_c_T = transpose(T_c_O);  
r_PT = [0;0;-R];
r_PTx = Vx([0;0;-R]);
O_w_T = [states(1);states(2);states(3)]; O_w_Tx =Vx(O_w_T);

O_vel_TO = Vx(O_c_T*O_w_T)*[0;0;R];
u_TO = O_vel_TO(1);
v_TO = O_vel_TO(2);

murr = mu0*tanh((u_TO^2 + v_TO^2)/v_thres); 
roll_rest_coeff = [1,0,-murr*u_TO/sqrt(u_TO^2 + v_TO^2);0,1,-murr*v_TO/sqrt(u_TO^2 + v_TO^2);0,0,1];
FG = [0;0;-(mf+6*m)*g];
FR  = -murr*norm(FG)/sqrt(u_TO^2 + v_TO^2)*[u_TO; v_TO; 0];

f3_u = zeros(3,1);
Amat = I_T + (mf + 6*m)*r_CMTx*T_c_O*r_PTx*O_c_T - m*r_m1Tx*r_m1Tx - m*r_m2Tx*r_m2Tx...
       - m*r_m3Tx*r_m3Tx - m*r_m4Tx*r_m4Tx - m*r_m5Tx*r_m5Tx - m*r_m6Tx*r_m6Tx...
       - (mf + 6*m)*Vx(T_c_O*r_PT)*Vx(T_c_O*r_PT) + (mf + 6*m)*Vx(T_c_O*r_PT)*r_CMTx;
  %some mistakes here. check again 
Bvec = -cross(O_w_T,I_T*O_w_T) - m*cross(r_m1T,2*O_w_Tx*T_v_m1T + O_w_Tx*O_w_Tx*r_m1T)...
       - m*r_m2Tx*(T_a_m2T + 2*O_w_Tx*T_v_m2T + O_w_Tx*O_w_Tx*r_m2T)...
       - m*r_m3Tx*(T_a_m3T + 2*O_w_Tx*T_v_m3T + O_w_Tx*O_w_Tx*r_m3T)...
       - m*r_m4Tx*(T_a_m4T + 2*O_w_Tx*T_v_m4T + O_w_Tx*O_w_Tx*r_m4T)...
       - m*r_m5Tx*(T_a_m5T + 2*O_w_Tx*T_v_m5T + O_w_Tx*O_w_Tx*r_m5T)...
       - m*r_m6Tx*(T_a_m6T + 2*O_w_Tx*T_v_m6T + O_w_Tx*O_w_Tx*r_m6T)...
       + r_CMTx*T_c_O*FG + (mf + 6*m)*cross(T_c_O*r_PT, T_a_CMT + ...
         2*O_w_Tx*T_v_CMT + O_w_Tx*O_w_Tx*r_CMT) - T_c_O*cross(r_PT, FG) ...
         - T_c_O*cross(r_PT, FW);%- T_c_O*cross(r_PT, FR);
f3_u = inv(Amat)*Bvec;
end

== matlab function comprehensive_model_with_rocks_trial/command filter based backstepper1/alpha calculator ==
  data: ref input size=3; alpha output size=3; ref_dot input; states input size=13; R parameter size=1; f1 output size=[3,3]; K1 output size=[3,3]
function [alpha, f1, K1] = alpha_calculator(ref, ref_dot, states, R)
q0 = states(10); q1 = states(11); q2 = states(12); q3 = states(13);

xc_dot = ref_dot;
xc = ref;
x = [states(7); states(8); states(9)];

K1 = 3*eye(3);

Rx = [0,R,0;-R,0,0;0,0,1];

T_c_O = [q0^2 + q1^2 - q2^2 - q3^2, 2*(q1*q2 + q0*q3), 2*(q1*q3 - q0*q2);...
2*(q1*q2 - q0*q3), q0^2 - q1^2 + q2^2 - q3^2, 2*(q2*q3 + q0*q1);...
2*(q1*q3 + q0*q2), 2*(q2*q3 - q0*q1), q0^2 - q1^2 - q2^2 + q3^2];
O_c_T = transpose(T_c_O);

f1 = Rx*O_c_T;
alpha = inv(f1)*(xc_dot - K1*(x - xc));
end

== matlab function comprehensive_model_with_rocks_trial/command filter based backstepper1/main one/MATLAB Function ==
  data: u input; f3_u output size=3; u_dot input; u_ddot input; states input; v_thres parameter; d parameter; R parameter; mu0 parameter; mf parameter; m parameter; Izz parameter; Iyy parameter; Ixx parameter; g parameter
function f3_u = f3u_calculator(u,u_dot,u_ddot,states,v_thres, d, R, mu0, mf, m, Izz, Iyy, Ixx, g)
I_T = [Ixx,0,0;0,Iyy,0;0,0,Izz];
r_m1T = [u(1);0;0];             T_v_m1T = [u_dot(1);0;0]; T_a_m1T = [u_ddot(1);0;0];
r_m2T = [-(d - u(1));0;0];      T_v_m2T = [u_dot(1);0;0]; T_a_m2T = [u_ddot(1);0;0];
r_m3T = [0;u(2);0];             T_v_m3T = [0;u_dot(2);0]; T_a_m3T = [0;u_ddot(2);0];
r_m4T = [0;-(d - u(2));0];      T_v_m4T = [0;u_dot(2);0]; T_a_m4T = [0;u_ddot(2);0];
r_m5T = [0;0;u(3)];             T_v_m5T = [0;0;u_dot(3)]; T_a_m5T = [0;0;u_ddot(3)];
r_m6T = [0;0;-(d - u(3))];      T_v_m6T = [0;0;u_dot(3)]; T_a_m6T = [0;0;u_ddot(3)];
r_CMT = m*(r_m1T + r_m2T + r_m3T + r_m4T + r_m5T + r_m6T)/(6*m+mf);
T_v_CMT = m*(T_v_m1T + T_v_m2T + T_v_m3T + T_v_m4T + T_v_m5T + T_v_m6T)/(6*m+mf);
T_a_CMT = m*(T_a_m1T + T_a_m2T + T_a_m3T + T_a_m4T + T_a_m5T + T_a_m6T)/(6*m+mf);
r_CMTx = Vx(r_CMT);r_m1Tx = Vx(r_m1T);r_m2Tx = Vx(r_m2T);r_m3Tx = Vx(r_m3T);
r_m4Tx = Vx(r_m4T);r_m5Tx = Vx(r_m5T);r_m6Tx = Vx(r_m6T);
q0 = states(10);q1=states(11);q2=states(12);q3=states(13);
T_c_O = [q0^2 + q1^2 - q2^2 - q3^2, 2*(q1*q2 + q0*q3), 2*(q1*q3 - q0*q2);...
       2*(q1*q2 - q0*q3), q0^2 - q1^2 + q2^2 - q3^2, 2*(q2*q3 + q0*q1);...
       2*(q1*q3 + q0*q2), 2*(q2*q3 - q0*q1), q0^2 - q1^2 - q2^2 + q3^2];
O_c_T = transpose(T_c_O);  
r_PT = [0;0;-R];
r_PTx = Vx([0;0;-R]);
O_w_T = [states(1);states(2);states(3)]; O_w_Tx =Vx(O_w_T);

O_vel_TO = Vx(O_c_T*O_w_T)*[0;0;R];
u_TO = O_vel_TO(1);
v_TO = O_vel_TO(2);

murr = mu0*tanh((u_TO^2 + v_TO^2)/v_thres); 
roll_rest_coeff = [1,0,-murr*u_TO/sqrt(u_TO^2 + v_TO^2);0,1,-murr*v_TO/sqrt(u_TO^2 + v_TO^2);0,0,1];
FG = [0;0;-(mf+6*m)*g];
FR  = -murr*norm(FG)/sqrt(u_TO^2 + v_TO^2)*[u_TO; v_TO; 0];

f3_u = zeros(3,1);
Amat = I_T + (mf + 6*m)*r_CMTx*T_c_O*r_PTx*O_c_T - m*r_m1Tx*r_m1Tx - m*r_m2Tx*r_m2Tx...
       - m*r_m3Tx*r_m3Tx - m*r_m4Tx*r_m4Tx - m*r_m5Tx*r_m5Tx - m*r_m6Tx*r_m6Tx...
       - (mf + 6*m)*Vx(T_c_O*r_PT)*Vx(T_c_O*r_PT) + (mf + 6*m)*Vx(T_c_O*r_PT)*r_CMTx;
  %some mistakes here. check again 
Bvec = -cross(O_w_T,I_T*O_w_T) - m*cross(r_m1T,2*O_w_Tx*T_v_m1T + O_w_Tx*O_w_Tx*r_m1T)...
       - m*r_m2Tx*(T_a_m2T + 2*O_w_Tx*T_v_m2T + O_w_Tx*O_w_Tx*r_m2T)...
       - m*r_m3Tx*(T_a_m3T + 2*O_w_Tx*T_v_m3T + O_w_Tx*O_w_Tx*r_m3T)...
       - m*r_m4Tx*(T_a_m4T + 2*O_w_Tx*T_v_m4T + O_w_Tx*O_w_Tx*r_m4T)...
       - m*r_m5Tx*(T_a_m5T + 2*O_w_Tx*T_v_m5T + O_w_Tx*O_w_Tx*r_m5T)...
       - m*r_m6Tx*(T_a_m6T + 2*O_w_Tx*T_v_m6T + O_w_Tx*O_w_Tx*r_m6T)...
       + r_CMTx*T_c_O*FG + (mf + 6*m)*cross(T_c_O*r_PT, T_a_CMT + ...
         2*O_w_Tx*T_v_CMT + O_w_Tx*O_w_Tx*r_CMT) - T_c_O*cross(r_PT, FG) ...
         ;%- T_c_O*cross(r_PT, FR);
f3_u = inv(Amat)*Bvec;
end

== matlab function comprehensive_model_with_rocks_trial/bouncing_model/rockfield_gen1/MATLAB Function1 ==
  data: t input; states input; rock_cents output; rock_cents input; rock_radi input; set_sig input; limit input; rock_radi output; set_sig output; limit output; all_rock_rads input; all_rock_cents input; R parameter
function [rock_cents,rock_radi,set_sig,limit]  = field_gen(t,states,rock_cents,rock_radi,set_sig,limit,  all_rock_rads,all_rock_cents, R)

if t== 0
    set_sig = 1;
    limit = 50;
    rock_cents = all_rock_cents(:,:,1);
    rock_radi = abs(all_rock_rads(1,:)).';
end
if (abs(states(7) - limit) < 1 && states(7) < limit && set_sig == 0) 
    exists_curr_rock = false;
    rock_cents_curr = [0;0;0];
    rock_radi_curr = 0;
    for i = 1:50
        if norm(states(7:9,1) - rock_cents(:,i)) <= abs(rock_radi(i,1)) + R + 0.001
            rock_cents_curr = rock_cents(:,i);
            rock_radi_curr = abs(rock_radi(i,1));
            exists_curr_rock = true;
            break;
        end
    end
        
    set_sig = 1;
    limit = limit + 50;
    rock_cents = all_rock_cents(:,:,limit/50);
    %rock_cents(3,:) = states(9) - min_dist*kA + (-0.2 + rockcent_rand(3,:)*(0.3));
    rock_radi = abs(all_rock_rads(limit/50,:)).';
    if exists_curr_rock
    rock_cents(:,i) = rock_cents_curr;
    rock_radi(i,1) = rock_radi_curr;
    end
else
    set_sig = 0;
end
% 
% set_sig = 0;
% limit = 0;
% rock_cents = [[32.4447642464399;6.15387066786823;0.0807251010000357],[27.1087651500054;5.98144588572040;-0.0993103008714087], [33;8;0]];
% rock_radi = [0.635767172476899;0.0922765736963689;0.4];
end

== matlab function comprehensive_model_with_rocks_trial/bouncing_model/rockfield_gen/MATLAB Function1 ==
  data: t input; states input; rock_cents output; rockcent_rand input; rockrad_rand input; rock_cents input; rock_radi input; set_sig input; limit input; rock_radi output; R parameter; set_sig output; limit output
function [rock_cents,rock_radi,set_sig,limit]  = field_gen(t,states,rockcent_rand,rockrad_rand,rock_cents,rock_radi,set_sig,limit,R)

if t== 0
    set_sig = 1;
    limit = 50;
    rock_cents(1,:) = 25 + rockcent_rand(1,:)*(25);
    rock_cents(2,:) = states(8) + (-25 +rockcent_rand(2,:)*(50));
    rock_cents(3,:) = states(9) -R + (-0.1 + rockcent_rand(3,:)*(0.2));
        rock_radi = abs(rockrad_rand(:,1));
end
if (abs(states(7) - limit) < 1 && states(7) < limit && set_sig == 0) 
    exists_curr_rock = false;
    rock_cents_curr = [0;0;0];
    rock_radi_curr = 0;
    curr_rock_ind = 0;
    for i = 1:50
        if norm(states(7:9,1) - rock_cents(:,i)) <= abs(rock_radi(i,1)) + R + 0.001
            rock_cents_curr = rock_cents(:,i);
            rock_radi_curr = abs(rock_radi(i,1));
            exists_curr_rock = true;
            curr_rock_ind = i;
            break;
        end
    end
        
    set_sig = 1;
    rock_cents(1,:) = limit + rockcent_rand(1,:)*(50);
    rock_cents(2,:) = states(8) + (-25 +rockcent_rand(2,:)*(50));
    rock_cents(3,:) =  (-0.1 + rockcent_rand(3,:)*(0.2));
    %rock_cents(3,:) = states(9) - min_dist*kA + (-0.2 + rockcent_rand(3,:)*(0.3));
    rock_radi = abs(rockrad_rand(:,1));

    for i = 1:50
        if rock_radi(i,1) <= 0.05
            rock_radi(i,1) = rock_radi(i,1)*10;
        end
        if (rock_cents(1,i) - rock_radi(i,1)) <= limit
            rock_cents(1,i) = rock_cents(1,i) + rock_radi(i,1);
        end
    end
    if exists_curr_rock
        rock_cents(:,curr_rock_ind) = rock_cents_curr;
        rock_radi(curr_rock_ind,1) = rock_radi_curr;
    end
    limit = limit + 50;
else
    set_sig = 0;
end
% 
% set_sig = 0;
% limit = 0;
% rock_cents = [[32.4447642464399;6.15387066786823;0.0807251010000357],[27.1087651500054;5.98144588572040;-0.0993103008714087], [33;8;0]];
% rock_radi = [0.635767172476899;0.0922765736963689;0.4];

end
